simulink model "PenduloSimple"  (R2024b)
settings: Solver=VariableStepAuto  StartTime=0.0  StopTime=10.0  RelTol=1e-3
settings Model: Creator=david  LastModifiedBy=david

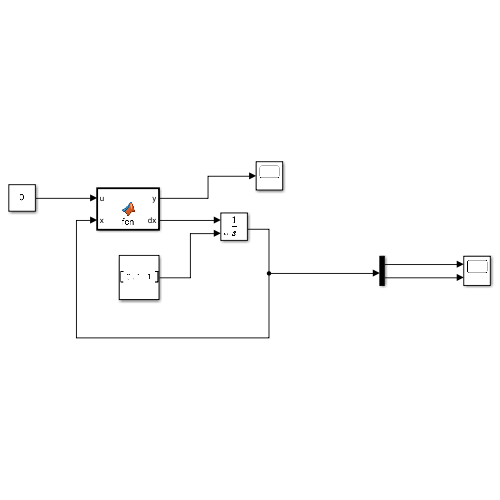
[thumbnail: Simulink's stored preview of the top-level diagram]
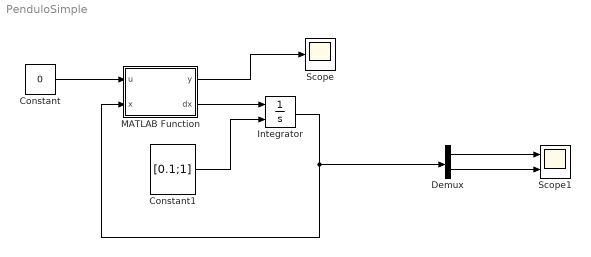
== system PenduloSimple ==
  Constant : Constant  Value=0
  Constant1 : Constant  Value=[0.1;1]
  Demux : Demux  Outputs=2
  Integrator : Integrator  InitialConditionSource=external
  MATLAB Function : MATLAB Function  TreatAsAtomicUnit=on
  Scope : Scope
  Scope1 : Scope  NumInputPorts=2
  wires:
  Constant/1 -> MATLAB Function/1(u)
  MATLAB Function/2(dx) -> Integrator/1
  Integrator/1 -> Demux/1, MATLAB Function/2(x)
  Constant1/1 -> Integrator/2
  MATLAB Function/1(y) -> Scope/1
  Demux/1 -> Scope1/1
  Demux/2 -> Scope1/2

== matlab function PenduloSimple/MATLAB Function ==
  data: y output; dx output; u input; x input
function [y, dx] = fcn(u, x)
g = 9.81;  
l = 1;     
m = 1;     
b = 0.5;   

x1 = x(1);  
x2 = x(2);  

dx1 = x2;
dx2 = -(g/l)*sin(x1) - (b/(m*l^2))*x2 + u/(m*l^2);

dx = [dx1; dx2];

y = x1;
